simulink model "IQ_Radio"  (R2019a)
settings: Solver=FixedStepAuto  StartTime=0.0  StopTime=10.0  RelTol=1e-3
libraries: simrfV2elements x4, simrfV2util1 x2, commrandsrc3 x2, simrfV2sources1 x2, simrfV2_lib x1
settings Model: Creator=owatkins  LastModifiedBy=owatkins

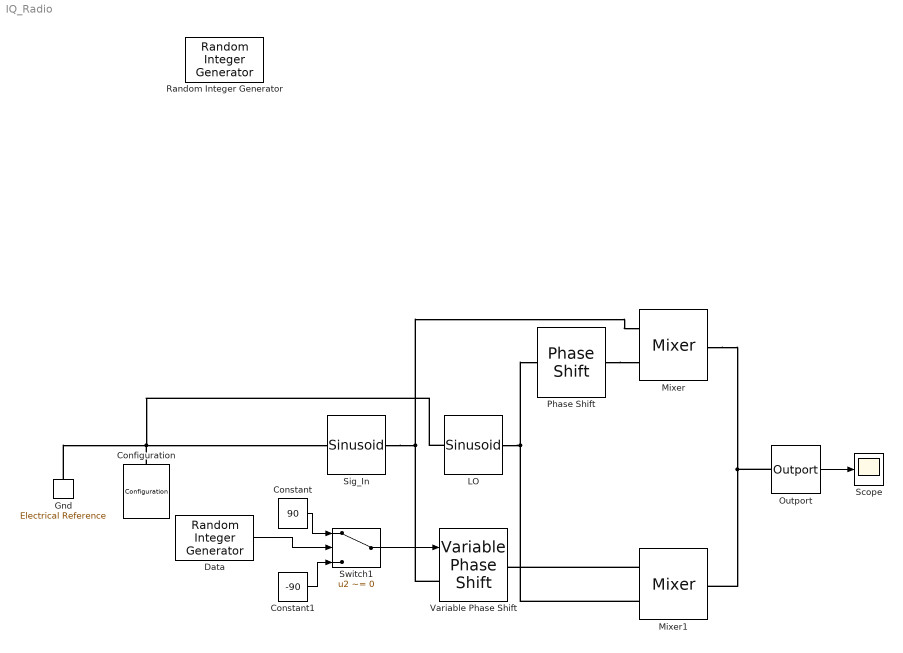
== system IQ_Radio ==
  Configuration : simrfV2util1/Configuration  AutoFreq=on  Tones=[] Hz  Harmonics=[]  NormalizeCarrierPower=on  SolverType=Auto  UseCCode=on  StepSize=1e-6 s  AddNoise=on  defaultRNG=on  Seed=0  Temperature=290.0 K  SolverDelFlag=0  AbsTol=1e-6  RelTol=1e-3  MaxIter=10  ErrorEstimationType=2-norm over all variables  EnableInterpFilter=on  HiddenFIRfilterControllerParam=off  SmallSignalApprox=off  AllSimFreqs=on  SimFreqs=[] Hz  SimFreqsInternal=[]
      settings: SourceProductName=RF Blockset  SourceProductBaseCode=RB
  Constant : Constant  Value=90
  Constant1 : Constant  Value=-90
  Data : commrandsrc3/Random Integer Generator  SetSize=1  SeedSource=Auto  Seed=0  SampleTime=1  SamplesPerFrame=1  OutputDataType=uint8  SimulateUsing=Interpreted execution
      settings: SourceProductName=Communications Toolbox
  Gnd : simrfV2_lib/Elements/Electrical Reference
      settings: SourceProductName=RF Blockset  SourceProductBaseCode=RB
  LO : simrfV2sources1/Sinusoid  SineSourceType=Ideal voltage  VO_I=0 V  IO_I=0 A  VO_Q=0 V  IO_Q=0 A  VA_I=1.8 V  IA_I=0 A  VA_Q=0 V  IA_Q=0 A  Fmod=0 Hz  TD=0 s  CarrierFreq=5 MHz  InternalGrounding=off
      settings: SourceProductName=RF Blockset  SourceProductBaseCode=RB
  Mixer : simrfV2elements/Mixer  classname=mixer  Source_linear_gain=Available power gain  linear_gain=0 dB  Zin=50  Zout=50  ZLO=inf  Source_Poly=Even and odd order  Poly_Coeffs=[0 1]  IPType=Output  IP2=Inf dBm  IP3=Inf dBm  P1dB=Inf dBm  Psat=Inf dBm  Gcomp=Inf dBm  NF=0  InternalGrounding=on
      settings: SourceProductName=RF Blockset  SourceProductBaseCode=RB
  Mixer1 : simrfV2elements/Mixer  classname=mixer  Source_linear_gain=Available power gain  linear_gain=0 dB  Zin=50  Zout=50  ZLO=inf  Source_Poly=Even and odd order  Poly_Coeffs=[0 1]  IPType=Output  IP2=Inf dBm  IP3=Inf dBm  P1dB=Inf dBm  Psat=Inf dBm  Gcomp=Inf dBm  NF=0  InternalGrounding=on
      settings: SourceProductName=RF Blockset  SourceProductBaseCode=RB
  Outport : simrfV2util1/Outport  SensorType=Ideal voltage  OutputFormat=Complex Baseband  CarrierFreq=0 Hz  ZL=Inf  InternalGrounding=on  StepSize=1e-6 s  AutoStep=on
      settings: SourceProductName=RF Blockset  SourceProductBaseCode=RB
  Phase Shift : simrfV2elements/Phase Shift  PhaseShift=90 deg  InternalGrounding=on
      settings: SourceProductName=RF Blockset  SourceProductBaseCode=RB
  Scope : Scope
  Sig_In : simrfV2sources1/Sinusoid  SineSourceType=Ideal voltage  VO_I=0 V  IO_I=0 A  VO_Q=0 V  IO_Q=0 A  VA_I=1.8 V  IA_I=0 A  VA_Q=0 V  IA_Q=0 A  Fmod=0 Hz  TD=0 s  CarrierFreq=10 kHz  InternalGrounding=off
      settings: SourceProductName=RF Blockset  SourceProductBaseCode=RB
  Switch1 : Switch  Criteria=u2 ~= 0
  Variable Phase Shift : simrfV2elements/Variable Phase Shift  classname=varphase  PhaseShift_unit=deg  SparamZ0=50  InternalGrounding=on
      settings: SourceProductName=RF Blockset  SourceProductBaseCode=RB
  Random Integer Generator : commrandsrc3/Random Integer Generator  IOType=siggen  SetSize=8  SeedSource=Auto  Seed=0  SampleTime=1  SamplesPerFrame=1  OutputDataType=double  SimulateUsing=Interpreted execution
      settings: SourceProductName=Communications Toolbox
  wires:
  Constant/1 -> Switch1/1
  Constant1/1 -> Switch1/3
  Switch1/1 -> Variable Phase Shift/1
  Data/1 -> Switch1/2
  Outport/1 -> Scope/1
  connections:
  Sig_In/LConn1 -- Variable Phase Shift/LConn1 -- Mixer/LConn1
  Mixer1/LConn1 -- Variable Phase Shift/RConn1
  Mixer/RConn1 -- Outport/LConn1 -- Mixer1/RConn1
  Gnd/LConn1 -- LO/RConn1 -- Configuration/LConn1 -- Sig_In/RConn1
  LO/LConn1 -- Mixer1/LConn2 -- Phase Shift/LConn1
  Phase Shift/RConn1 -- Mixer/LConn2
